simulink model "ParameterIdentification"  (R2024b)
settings: Solver=FixedStepAuto  StartTime=0.0  StopTime=3  FixedStep=1e-6  MaxStep=1e-6  RelTol=1e-3
undefined symbols (not defined in the file): F1, Period, Pn, Ts, U_ref, Udc
libraries: My_library x3, spsDCVoltageSourceLib x1, spsGroundLib x1, simulink x1, spsPermanentMagnetSynchronousMachineLib x1, spsTwoLevelConverterLib x1, sps_lib x1
(part 2 of 2)

== matlab function ParameterIdentification/Subsystem/Sensorless/Subsystem/Flux&J_Identification/SVPWM_120 ==
  data: U_alpha input; Tcm1 output; U_beta input; Period input; U_dc input; Tcm2 output; Tcm3 output
function [Tcm1, Tcm2, Tcm3] = fcn(U_alpha, U_beta, Period, U_dc)
    % 计算 Tx, Ty
    scaleFactor = -sqrt(3) * Period / 2 / U_dc;
    Tx = scaleFactor * (sqrt(3) * 0.5 * U_alpha + 0.5 * U_beta);
    Ty = scaleFactor * U_beta;

    % 计算 Ta, Tb, Tc
    if Tx >= 0 && Ty >= 0
        Tc = 0;
        [Ta, Tb] = myfun(Tx, Ty, Period);
    elseif Tx <= Ty && Tx <= 0
        Ta = 0;
        [Tb, Tc] = myfun(Ty - Tx, -Tx, Period);
    elseif Tx > Ty && Ty <= 0
        Tb = 0;
        [Ta, Tc] = myfun(Tx - Ty, -Ty, Period);
    else
        error('Both Tx and Ty cannot be less than 0');
    end

    % 计算 T0
    T_max = max([Ta, Tb, Tc]);
    T0 = Period / 2 - T_max;

    % 计算 Tcm1, Tcm2, Tcm3
    Tcm1 = Ta + T0 / 2;
    Tcm2 = Tb + T0 / 2;
    Tcm3 = Tc + T0 / 2;

    % Tcm2 = Ta + T0 / 2;
    % Tcm3 = Tb + T0 / 2;
    % Tcm1 = Tc + T0 / 2;
end

function [T1, T2] = myfun(T3, T4, Period)
    T3_abs = abs(T3);
    T4_abs = abs(T4);
    halfPeriod = Period / 2;

    if T3_abs <= halfPeriod && T4_abs <= halfPeriod
        T1 = T3;
        T2 = T4;
    elseif T3_abs >= halfPeriod && T4_abs >= halfPeriod
        T1 = halfPeriod;
        T2 = halfPeriod;
    elseif T3_abs >= T4_abs
        if T3_abs - T4_abs >= halfPeriod
            T1 = halfPeriod;
            T2 = 0;
        else
            T1 = halfPeriod;
            T2 = halfPeriod * T4 / T3;
        end
    else
        if T4_abs - T3_abs >= halfPeriod
            T1 = 0;
            T2 = halfPeriod;
        else
            T1 = halfPeriod * T3 / T4;
            T2 = halfPeriod;
        end
    end
end

== matlab function ParameterIdentification/Subsystem/Sensorless/Subsystem/Flux&J_Identification/Id = 0/Subsystem4/MATLAB Function ==
  data: error input; output output; Kp input; Ki input; Kd input; Ts input; max_Integral input; min_Integral input; max_output input; min_output input
function output = fcn(error, Kp, Ki, Kd, Ts, max_Integral, min_Integral, max_output, min_output)
%定义参数
persistent last_error;
persistent I;

% 初始化静态变量（仅在第一次调用时执行）
if isempty(last_error)
last_error = 0;  % 假设初始误差为0
end
if isempty(I)
I = 0;           % 假设初始积分项为0
end

%比例项
P = Kp*error;

%积分项
I = I + Ki*error*Ts;
%积分限幅
if(I>=max_Integral)
    I = max_Integral;
elseif(I<=min_Integral)
    I = min_Integral;
end

%微分项
D = Kd*(error - last_error)/Ts;

%保留此次错误值
last_error = error;

%输出限幅
output = P+I+D;
if(output>=max_output)
    output = max_output;
elseif(output<=min_output)
    output = min_output;
end
